simulink subsystem "EKF"  (R2024a)
settings: Solver=VariableStepAuto  StartTime=0.0  StopTime=10.0  RelTol=1e-3
settings Model: Creator=Bocchio  LastModifiedBy=Bocchio

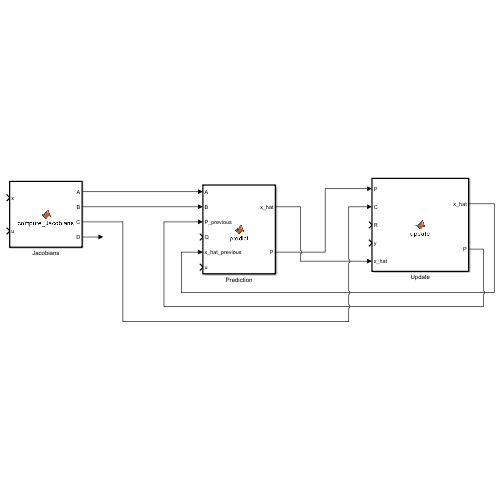
[thumbnail: Simulink's stored preview of the top-level diagram]
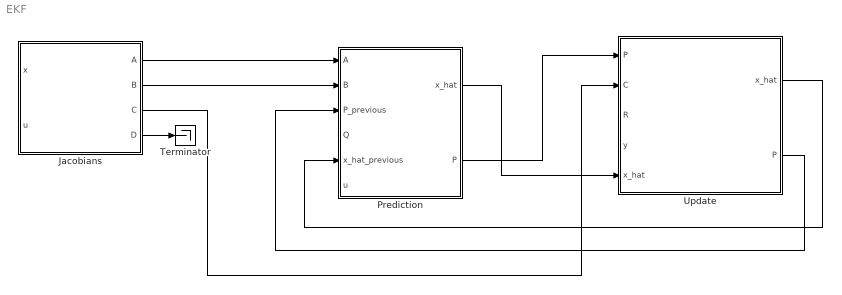
== system EKF ==
  Jacobians : MATLAB Function  TreatAsAtomicUnit=on
  Prediction : MATLAB Function  TreatAsAtomicUnit=on
  Terminator : Terminator
  Update : MATLAB Function  TreatAsAtomicUnit=on
  wires:
  Jacobians/1(A) -> Prediction/1(A)
  Jacobians/2(B) -> Prediction/2(B)
  Jacobians/4(D) -> Terminator/1
  Prediction/2(P) -> Update/1("P ")
  Jacobians/3(C) -> Update/2(C)
  Prediction/1(x_hat) -> Update/5("x_hat ")
  Update/2(P) -> Prediction/3(P_previous)
  Update/1(x_hat) -> Prediction/5(x_hat_previous)

== matlab function EKF/Prediction ==
  data: A input; B input; P_previous input; Q input; x_hat_previous input; u input; x_hat output; P output
function [x_hat, P] = predict(A, B, P_previous, Q, x_hat_previous, u)

x_hat = A * x_hat_previous + B * u;
P = A*P_previous*A' + Q;

end

== matlab function EKF/Jacobians ==
  data: x input; u input; A output; B output; C output; D output
function [A, B, C, D] = compute_Jacobians(x, u)

%% Parameters

% Physical constants
g   = 9.81; %[m/s^2]

% Structure
H = 98.00 * 1e-3; %[m]

% Ball/object
m = 60.54 * 1e-3;   %[kg]
r = 61.25/2 * 1e-3; %[m]


%% Drag related coefficients
rho = 1.21; %[kg/m^3]
Cd  = 0.45; %[Ns/m]


%% Current model
V1min = 4.300000e-02; %[V]
V2min = 4.300000e-02; %[V]
I1min = 2.383122e-02; %[A]
I2min = 2.591441e-02; %[A]
k1 = +1.165800e+01; %[V/MU]
k2 = +1.165800e+01; %[V/MU]
c1 = -5.608000e-01; %[V]
c2 = -5.608000e-01; %[V]


%% Inductances
% L(z, I) = L0 + Lz * exp(-az * z) + LI * atan(aI * I - bI);

% Static
L10 = 6.122809e-02; %[H]
L20 = 6.122809e-02; %[H]

% Position z
a1z = 1.837302e+02; %[1/m]
a2z = 1.837302e+02; %[1/m]
L1z = 3.438228e-02; %[H]
L2z = 3.438228e-02; %[H]

% Current I
a1I = 4.759750e+00; %[]
a2I = 4.759750e+00; %[]
b1I = 6.704755e-01; %[A]
b2I = 6.704755e-01; %[A]
L1I = 3.831209e-02; %[H]
L2I = 3.831209e-02; %[H]


%% Resistances
% R() = R0

% Static
R10 = 4.17; %[ohm]
R20 = 4.20; %[ohm]


%% Matrices

L1 = @(x, I) L10 + L1z * exp(-a1z*x) + L1I * atan(a1I * I - b1I);
L2 = @(x, I) L20 + L2z * exp(-a2z*(H - 2*r - x)) + L2I * atan(a2I * I - b2I);
dL1dx = @(x) -a1z*L1z * exp(-a1z*x);
dL2dx = @(x) +a2z*L2z * exp(-a2z*(H - 2*r - x));
dL1ddx = @(x) +a1z^2*L1z * exp(-a1z*x);
dL2ddx = @(x) +a2z^2*L2z * exp(-a2z*(H - 2*r - x));
% dL1dI = @(I) a1I * I / (1 + (a1I * I - b1I)^2);
% dL2dI = @(I) a2I * I / (1 + (a2I * I - b2I)^2);
% dL1ddI = @(I) -a1I * I / ((1 + (a1I * I - b1I)^2)^2 * 2*(a1I * I - b1I) * a1I);
% dL2ddI = @(I) -a2I * I / ((1 + (a2I * I - b2I)^2)^2 * 2*(a2I * I - b2I) * a2I);


% A coefficients
a11 = 0;
a12 = 1;
a13 = 0;
a14 = 0;

a21 = 1 / m * (1/2 * dL1ddx(x(1)) * x(3)^2 + 1/2 * dL2ddx(x(1)) * x(4)^2);
a22 = 0;
a23 = 1/m * dL1dx(x(1)) * x(3);
a24 = 1/m * dL2dx(x(1)) * x(4);

a31 = -1 / L1(x(1), x(3))^2 * dL1dx(x(1)) * (-R10 * x(3) + U_to_V(u(1)));
a32 = 0;
a33 = 1 / L1(x(1), x(3)) * (-R10);
a34 = 0;

a41 = -1 / L2(x(1), x(4))^2 * dL2dx(x(1)) * (-R20 * x(4) + U_to_V(u(2)));
a42 = 0;
a43 = 0;
a44 = 1 / L2(x(1), x(4)) * (-R20);

% B coefficients
b11 = 0;
b12 = 0;
b21 = 0;
b22 = 0;
b31 = 1 / L1(x(1), x(3)) * k1;
b32 = 0;
b41 = 0;
b42 = 1 / L2(x(1), x(4)) * k2;

% C coefficients
c1 = 1;
c2 = 0;
c3 = 0;
c4 = 0;

% D coefficients
d1 = 0;
d2 = 0;


% State matrices
A = [
    a11 a12 a13 a14;
    a21 a22 a23 a24;
    a31 a32 a33 a34;
    a41 a42 a43 a44
    ];

B = [
    b11 b12;
    b21 b22;
    b31 b32;
    b41 b42
    ];

C = [c1 c2 c3 c4];

D = [d1 d2];

end

== matlab function EKF/Update ==
  data: P input; x_hat output; C input; R input; y input; x_hat input; P output
function [x_hat, P] = update(P, C, R, y, x_hat)

K = (C .* P .* C' + R) \ (P .* C');
x_hat = x_hat + K * (y - C * x_hat);
P = (eye(size(P, 1)) - K*C) * P;

end
